simulink model "LinksMotorFahrplan"  (R2012b)
settings: Solver=FixedStepDiscrete  StartTime=0.0  StopTime=25  RelTol=1e-3
libraries: commutil2 x12, c280xlib x3, idelinklib_tgtpref x2, c2833xlib x1
settings Model: Creator=mit064  LastModifiedBy=mit064
settings DataIOCC: SaveOutput=off  SaveTime=off
settings OptimizationCC: OptimizeModelRefInitCode=on  LifeSpan=1
settings HardwareCC: ProdBitPerChar=16  ProdBitPerInt=16  ProdBitPerPointer=16  ProdLargestAtomicInteger=Integer  ProdIntDivRoundTo=Zero  ProdEndianess=LittleEndian  ProdWordSize=16  ProdHWDeviceType=Texas Instruments->C2000
settings RTWCC: SystemTargetFile=idelink_ert.tlc  GenerateMakefile=off  TemplateMakefile=none  Description=IDE Link ERT  ProcessScript=idelink_ert_make_rtw_hook
settings CodeAppCC: IgnoreCustomStorageClasses=off

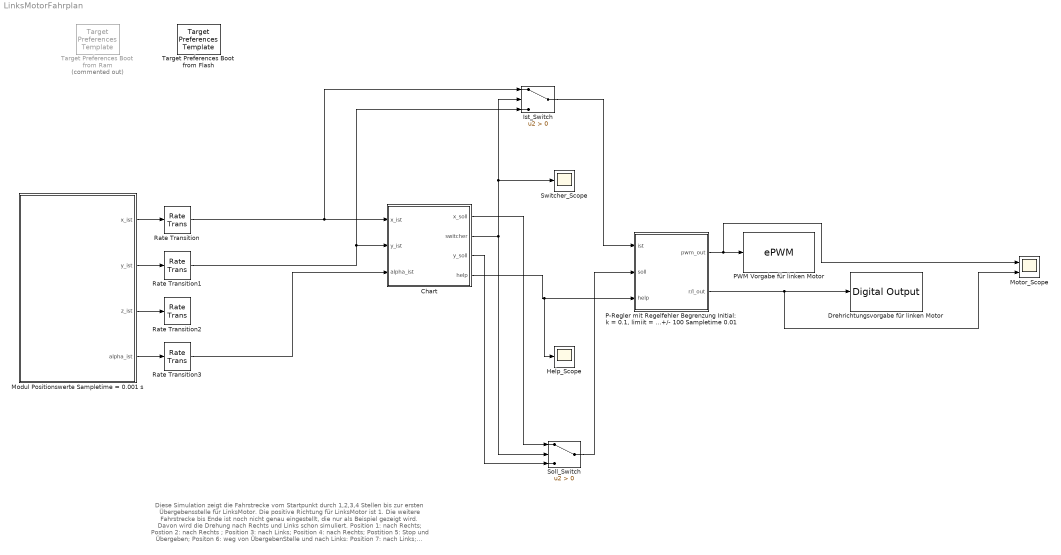
== system LinksMotorFahrplan ==
  note: Diese Simulation zeigt die Fahrstrecke vom Startpunkt durch 1,2,3,4 Stellen bis zur ersten Übergebensstelle für LinksMotor.
      | Die positive Richtung für LinksMotor ist 1.
      | Die weitere Fahrstrecke bis Ende ist noch nicht genau eingestellt, die nur als Beispiel gezeigt wird.
      | Davon wird die Drehung nach Rechts und Links schon simuliert.
      |
      | Position 1: nach Rechts; Postion 2: nach Rechts ; Position 3: nach Links; Position 4: nach Rechts;
      |  Postition 5: Stop und Übergeben; Positon 6: weg von ÜbergebenStelle und nach Links:
      | Position 7: nach Links; Postition 8: nach Links; Position 9: nach Links; Position 10 nach Links
      | Position 11: Stop und Übergeben, Position 12 Stop und Ende
      |
      | Prinzip der Chart:
      | 1. Eingänge: die x_ist, y_ist,alpha_ist Werte werden vom Nexoner Sensor ausgelesen.
      | Durch den Parameter Switcher nimmt der P-Regler die benötige x oder y Werte an.
      | 2. Ausgänge: Durch die Parameter Switcher nimmt ebenfalls der P-Regler die benötige x oder y Werte an.
      | 3. Parameter help in Ausgang: im Fall wenn der Fahrzeug sich nach Links umdrehen will, und  y_soll oder x_soll werte kleiner als den letzen Stelle ist,
      | wird "help" gleich eins, somit dreht sich der Linksmotor in negative Richtung .
      | 4. Parameter help in P-Regler: wenn help gleich eins ist, wird der Motor sich  immer in eine Richtung drehen.
  Chart : Stateflow chart  TreatAsAtomicUnit=on
  Drehrichtungsvorgabe für linken Motor : c2833xlib/Digital Output  GPIO_Number=GPIO16~GPIO23  GPIO_Bit0=off  GPIO_BIT0_Toggle=off  GPIO_Bit1=off  GPIO_BIT1_Toggle=off  GPIO_Bit2=off  GPIO_BIT2_Toggle=off  GPIO_Bit3=off  GPIO_BIT3_Toggle=off  GPIO_Bit4=off  GPIO_BIT4_Toggle=off  GPIO_Bit5=on  GPIO_BIT5_Toggle=off  GPIO_Bit6=off  GPIO_BIT6_Toggle=off  GPIO_Bit7=off  GPIO_BIT7_Toggle=off
  Help_Scope : Scope
  Ist_Switch : Switch  Criteria=u2 > Threshold
  Modul Positionswerte Sampletime = 0.001 s : Subsystem
  Motor_Scope : Scope  NumInputPorts=2
      settings: YMin=-5~-5  YMax=5~5  SaveName=ScopeData2
  "P-Regler mit Regelfehler Begrenzung Initial: k = 0.1, limiit = +/- 100 Sampletime 0.01" : Subsystem
  "PWM Vorgabe für linken Motor " : c280xlib/ePWM  checkMode=off  useModule=ePWM2  periodUnits=Clock cycles  timerSource=Specify via dialog  timerPeriod_clk=64000  timerPeriod_sec=0.0001  countingMode=Up  synchronizationOption=Disable  synchronizationEnable=off  phaseActiveEnable=Disable  phaseDirection=Count down after sync  phaseActive=0  clockPrescale=1  HSclockPrescale=1  ePWMxAStatus=off  CMPAUnits=Clock cycles  CMPASource=Specify via dialog  CMPAValue_per=50  CMPAValue_clk=32000  ePWMxAactionLogic1=Do nothing  ePWMxAactionLogic2=Clear  ePWMxAactionLogic3=Set  ePWMxAactionLogic4=Do nothing  ePWMxAactionLogic5=Do nothing  ePWMxAactionLogic6=Do nothing  ePWMxALoadMode=Load on CTR=Zero  ePWMxACSFenable=off  ePWMxACSFvalue=Forcing Disable  ePWMxASFreload=Zero  enHRPWM=off  HRPWM_LoadMode=CTR=ZERO  HRPWM_CTLMode=Phase control mode  HRPWM_EDGMode=Both edge  enSFO=on  ePWMxBStatus=on  CMPBUnits=Percentages  CMPBSource=Input port  CMPBValue_per=0  CMPBValue_clk=32000  ePWMxBactionLogic1=Do nothing  ePWMxBactionLogic2=Set  ePWMxBactionLogic3=Do nothing  ePWMxBactionLogic4=Do nothing  ePWMxBactionLogic5=Clear  ePWMxBactionLogic6=Do nothing  ePWMxBLoadMode=Load on CTR=Zero  ePWMxBCSFenable=off  ePWMxBCSFvalue=Forcing Disable  ePWMxBSFreload=Zero  enableDBePWMxA=off  enableDBePWMxB=off  DBpolarity=AH  DBedgeDelay=Positive  DBSource_ePWMxA=ePWMxA  DBSource_ePWMxB=ePWMxA  DBperiodSource=Specify via dialog  REDperiod=0  FEDperiod=0  adcstartModuleA=off  adcrequestEventA=First event  adcstartEventA=CTR=Zero  adcstartModuleB=off  adcrequestEventB=First event  adcstartEventB=CTR=Zero  intEn=off  intPrd=First event  intSel=CTR=Zero  chopperEnable=off  chopperFrequency=1  chopperFirstwidth=1  chopperDuty=12.5%  tripZonesource=Specify via dialog  tzselOSHT1=off  tzselOSHT2=off  tzselOSHT3=off  tzselOSHT4=off  tzselOSHT5=off  tzselOSHT6=off  tzselCBC1=off  tzselCBC2=off  tzselCBC3=off  tzselCBC4=off  tzselCBC5=off  tzselCBC6=off  enTzOstIntr=off  enTzCbcIntr=off  ePWMxAforced=No action  ePWMxBforced=No action  timerPeriod=-1  ePWMxAValue=0  ePWMxBValue=0  tripZoneoption=OSHT
  Rate Transition{,1..3} (4 alike) : RateTransition  OutPortSampleTime=0.01
  Soll_Switch : Switch  Criteria=u2 > Threshold
  Switcher_Scope : Scope
  Target Preferences Boot from Flash : idelinklib_tgtpref/Target Preferences Template  Tag=ccslinktgtpref_ccsv4  library=off
  Target Preferences Boot from Ram : idelinklib_tgtpref/Target Preferences Template  Tag=ccslinktgtpref_ccsv4  Commented=on  library=off
  wires:
  "P-Regler mit Regelfehler Begrenzung Initial: k = 0.1, limiit = +/- 100 Sampletime 0.01"/2(r/l_out) -> Motor_Scope/2, Drehrichtungsvorgabe für linken Motor/1
  "P-Regler mit Regelfehler Begrenzung Initial: k = 0.1, limiit = +/- 100 Sampletime 0.01"/1(pwm_out) -> Motor_Scope/1, "PWM Vorgabe für linken Motor "/1
  Ist_Switch/1 -> "P-Regler mit Regelfehler Begrenzung Initial: k = 0.1, limiit = +/- 100 Sampletime 0.01"/1(ist)
  Soll_Switch/1 -> "P-Regler mit Regelfehler Begrenzung Initial: k = 0.1, limiit = +/- 100 Sampletime 0.01"/2(soll)
  Chart/2(switcher) -> Soll_Switch/2, Switcher_Scope/1, Ist_Switch/2
  Chart/1(x_soll) -> Soll_Switch/1
  Chart/3(y_soll) -> Soll_Switch/3
  Chart/4(help) -> Help_Scope/1, "P-Regler mit Regelfehler Begrenzung Initial: k = 0.1, limiit = +/- 100 Sampletime 0.01"/3(help)
  Rate Transition/1 -> Chart/1(x_ist), Ist_Switch/1
  Rate Transition1/1 -> Chart/2(y_ist), Ist_Switch/3
  Rate Transition3/1 -> Chart/3(alpha_ist)
  Modul Positionswerte Sampletime = 0.001 s/1(x_ist) -> Rate Transition/1
  Modul Positionswerte Sampletime = 0.001 s/4(alpha_ist) -> Rate Transition3/1
  Modul Positionswerte Sampletime = 0.001 s/3(z_ist) -> Rate Transition2/1
  Modul Positionswerte Sampletime = 0.001 s/2(y_ist) -> Rate Transition1/1

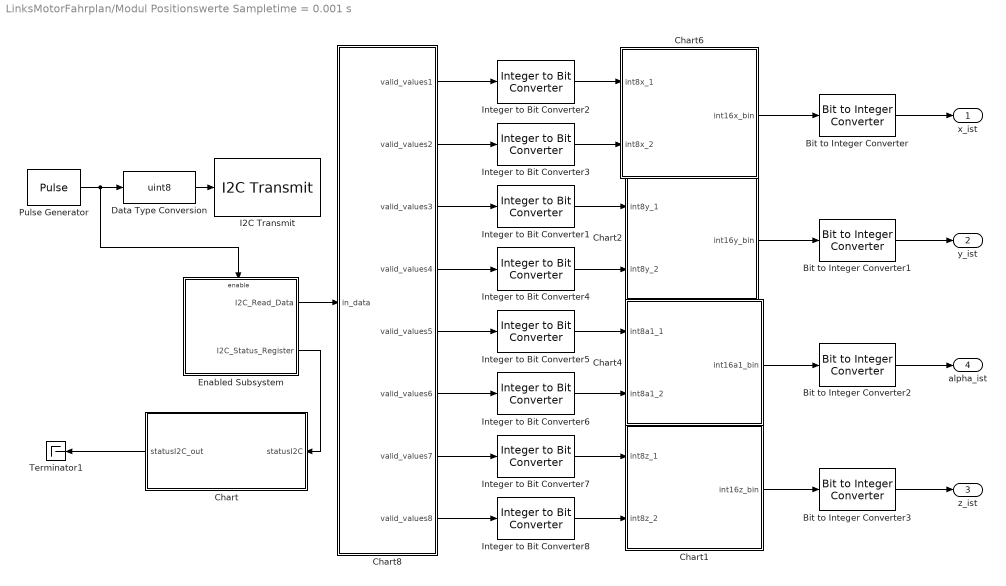
== system LinksMotorFahrplan/Modul Positionswerte Sampletime = 0.001 s ==
  Bit to Integer Converter{,1..3} (4 alike) : commutil2/Bit to Integer Converter  nbits=16  bitOrder=MSB first  signedOutputValues=Signed  outDtype=Inherit via internal rule  outDtypeSigned=Inherit via internal rule
  Chart : Stateflow chart  TreatAsAtomicUnit=on
  Chart1 : Stateflow chart  TreatAsAtomicUnit=on
  Chart2 : Stateflow chart  TreatAsAtomicUnit=on
  Chart4 : Stateflow chart  TreatAsAtomicUnit=on
  Chart6 : Stateflow chart  TreatAsAtomicUnit=on
  Chart8 : Stateflow chart  TreatAsAtomicUnit=on
  Data Type Conversion : DataTypeConversion  OutDataTypeStr=uint8
  Enabled Subsystem : Subsystem  TreatAsAtomicUnit=on
  I2C Transmit : c280xlib/I2C Transmit  addrFormat=7-Bit addressing  saSource=Specify via dialog  SAR=80  bitCount=8  STP=off  RM=off  STR=off
  Integer to Bit Converter{1..8} (8 alike) : commutil2/Integer to Bit Converter  nbits=8  signedInputValues=Unsigned  bitOrder=MSB first  outDtype=uint8
  Pulse Generator : DiscretePulseGenerator  Period=250  PulseWidth=249  SampleTime=0.001
  Terminator1 : Terminator
  x_ist : Outport
  y_ist : Outport  Port=2
  z_ist : Outport  Port=3
  alpha_ist : Outport  Port=4
  wires:
  Chart8/5(valid_values5) -> Integer to Bit Converter5/1
  Chart8/2(valid_values2) -> Integer to Bit Converter3/1
  Chart8/4(valid_values4) -> Integer to Bit Converter4/1
  Chart2/1(int16y_bin) -> Bit to Integer Converter1/1
  Chart8/1(valid_values1) -> Integer to Bit Converter2/1
  Chart8/3(valid_values3) -> Integer to Bit Converter1/1
  Integer to Bit Converter3/1 -> Chart6/2(int8x_2)
  Chart6/1(int16x_bin) -> Bit to Integer Converter/1
  Integer to Bit Converter1/1 -> Chart2/1(int8y_1)
  Integer to Bit Converter2/1 -> Chart6/1(int8x_1)
  Integer to Bit Converter4/1 -> Chart2/2(int8y_2)
  Bit to Integer Converter1/1 -> y_ist/1
  Integer to Bit Converter5/1 -> Chart4/1(int8a1_1)
  Integer to Bit Converter6/1 -> Chart4/2(int8a1_2)
  Bit to Integer Converter/1 -> x_ist/1
  Bit to Integer Converter2/1 -> alpha_ist/1
  Chart8/6(valid_values6) -> Integer to Bit Converter6/1
  Chart4/1(int16a1_bin) -> Bit to Integer Converter2/1
  Chart1/1(int16z_bin) -> Bit to Integer Converter3/1
  Enabled Subsystem/1(I2C_Read_Data) -> Chart8/1(in_data)
  Bit to Integer Converter3/1 -> z_ist/1
  Chart8/8(valid_values8) -> Integer to Bit Converter8/1
  Chart8/7(valid_values7) -> Integer to Bit Converter7/1
  Integer to Bit Converter8/1 -> Chart1/2(int8z_2)
  Integer to Bit Converter7/1 -> Chart1/1(int8z_1)
  Enabled Subsystem/2(I2C_Status_Register) -> Chart/1(statusI2C)
  Chart/1(statusI2C_out) -> Terminator1/1
  Pulse Generator/1 -> Enabled Subsystem/Enable, Data Type Conversion/1
  Data Type Conversion/1 -> I2C Transmit/1

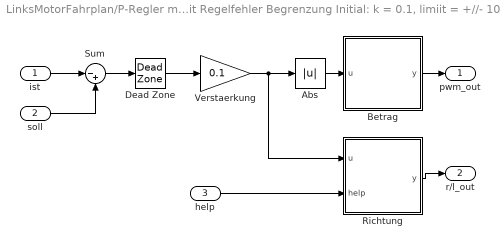
== system LinksMotorFahrplan/P-Regler mit Regelfehler Begrenzung Initial: k = 0.1, limiit = +//- 100 Sampletime 0.01 ==
  ist : Inport
  soll : Inport  Port=2
  help : Inport  Port=3
  Abs : Abs  SampleTime=0.01
  Betrag : MATLAB Function  TreatAsAtomicUnit=on  SystemSampleTime=0.01
  Dead Zone : DeadZone  LowerValue=-100  UpperValue=100  SampleTime=0.01  SaturateOnIntegerOverflow=on
  Richtung : MATLAB Function  TreatAsAtomicUnit=on  SystemSampleTime=0.01
  Sum : Sum  Inputs=|-+  SampleTime=0.01
  Verstaerkung : Gain  Gain=0.1  SampleTime=0.01
  pwm_out : Outport
  r/l_out : Outport  Port=2
  wires:
  Betrag/1(y) -> pwm_out/1
  Sum/1 -> Dead Zone/1
  Verstaerkung/1 -> Abs/1, Richtung/1(u)
  Dead Zone/1 -> Verstaerkung/1
  Abs/1 -> Betrag/1(u)
  soll/1 -> Sum/2
  Richtung/1(y) -> r/l_out/1
  ist/1 -> Sum/1
  help/1 -> Richtung/2(help)

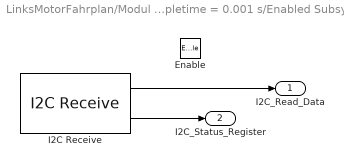
== system LinksMotorFahrplan/Modul Positionswerte Sampletime = 0.001 s/Enabled Subsystem ==
  Enable : EnablePort  StatesWhenEnabling=reset
  I2C Receive : c280xlib/I2C Receive  addrFormat=7-Bit addressing  saSource=Specify via dialog  SAR=80  bitCount=8  dataLength=10  initValue=0  NACK=on  STP=off  STR=on  sampleTime=0.001  dataType=uint8
  I2C_Read_Data : Outport
  I2C_Status_Register : Outport  Port=2
  wires:
  I2C Receive/2 -> I2C_Status_Register/1
  I2C Receive/1 -> I2C_Read_Data/1

== stateflow chart LinksMotorFahrplan/Modul Positionswerte Sampletime = 0.001 s/Chart1 ==
  state Daten_einlesen
  state x0
  state x1_1
    int16z_bin[0] = int8z_1[0];
    int16z_bin[1] = int8z_1[1];
    int16z_bin[2] = int8z_1[2];
    int16z_bin[3] = int8z_1[3];
    int16z_bin[4] = int8z_1[4];
    int16z_bin[5] = int8z_1[5]
    int16z_bin[6] = int8z_1[6];
    int16z_bin[7] = int8z_1[7];
    int16z_bin[8] = int8z_2[0];
    int16z_bin[9] = int8z_2[1];
    int16z_bin[10] = int8z_2[2];
    int16z_bin[11] = int8z_2[3];
    int16z_bin[12] = int8z_2[4];
    int16z_bin[13] = int8z_2[5]
    int16z_bin[14] = int8z_2[6];
    int16z_bin[15] = int8z_2[7];
  x0 -> Daten_einlesen
  (default) -> x0
  Daten_einlesen -> x1_1
  x1_1 -> Daten_einlesen
  data: int8z_1 input size=8; int8z_2 input size=8; int16z_bin output size=16 =0

== stateflow chart LinksMotorFahrplan/Chart ==
  state Start
  state Position_3
    switcher=0;
    help=1;
    state Position_3
      entry:y_soll=400;
    state Stop
      entry:y_soll=y_ist;
      exit:help=0;
    state Drehen_Linke
      entry:y_soll=0;
      exit:help=0;
    state stop
      entry:y_soll=y_ist;
    (default) -> Position_3.Position_3
    Position_3.Position_3 -> Position_3.Stop : [y_ist<402&&y_ist>398]
    Position_3.Stop -> Position_3.Drehen_Linke : [after(1,sec)]
    Position_3.Drehen_Linke -> Position_3.stop : [alpha_ist<65&&alpha_ist>61]
  state Position_4
    switcher=0;
    help=1;
    state Position_4
      entry:y_soll=700;
    state Stop
      entry:y_soll=y_ist;
    state Drehen_Recht
      entry:y_soll=0;
    state stop
      entry:y_soll=y_ist;
    (default) -> Position_4.Position_4
    Position_4.Position_4 -> Position_4.Stop : [y_ist<702&&y_ist>698]
    Position_4.Stop -> Position_4.Drehen_Recht : [after(1,sec)]
    Position_4.Drehen_Recht -> Position_4.stop : [alpha_ist<-61&&alpha_ist>-65]
  state Position_1
    switcher=0;
    help=1;
    state Position_1
      entry:y_soll=350;
    state Stop
      entry:y_soll=y_ist;
    state Drehen_Recht
      entry:y_soll=0;
    state stop
      entry:y_soll=y_ist;
    (default) -> Position_1.Position_1
    Position_1.Position_1 -> Position_1.Stop : [y_ist<352&&y_ist>348]
    Position_1.Stop -> Position_1.Drehen_Recht : [after(1,sec)]
    Position_1.Drehen_Recht -> Position_1.stop : [alpha_ist<79&&alpha_ist>75]
  state Position_2
    switcher=0;
    help=1;
    state Position_2
      entry:y_soll=900;
    state Stop
      entry:y_soll=y_ist;
    state Drehen_Recht
      entry:y_soll=0;
    state stop
      entry:y_soll=y_ist;
    (default) -> Position_2.Position_2
    Position_2.Position_2 -> Position_2.Stop : [y_ist<902&&y_ist>898]
    Position_2.Stop -> Position_2.Drehen_Recht : [after(1,sec)]
    Position_2.Drehen_Recht -> Position_2.stop : [alpha_ist>-61&&alpha_ist<-57]
  state Position_6
    switcher=0;
    help=1;
    state Position_6
      entry:y_soll=300;
    state Stop
      entry:y_soll=y_ist;
      exit:help=0;
    state Drehen_Linke
      entry:y_soll=0;
      exit:help=0;
    state stop
      entry:y_soll=y_ist;
    (default) -> Position_6.Position_6
    Position_6.Position_6 -> Position_6.Stop : [y_ist<302&&y_ist>298]
    Position_6.Stop -> Position_6.Drehen_Linke : [after(1,sec)]
    Position_6.Drehen_Linke -> Position_6.stop : [alpha_ist<-32&&alpha_ist>-36]
  state Position_5_give
    switcher=0;
    help=1;
    state Position_5
      entry:y_soll=400;
    state Stop
      entry:y_soll=y_ist;
    state Drehen_Recht
      entry:y_soll=0;
    state stop
      entry:y_soll=y_ist;
    (default) -> Position_5
    Position_5 -> Position_5_give.Stop : [y_ist<402&&y_ist>398]
    Position_5_give.Stop -> Position_5_give.Drehen_Recht : [after(5,sec)]
    Position_5_give.Drehen_Recht -> Position_5_give.stop : [alpha_ist<-88]
  state Position_7
    switcher=1;
    help=1;
    state Position_7
      entry:x_soll=1400;
    state Stop
      entry:x_soll=x_ist;
      exit:help=0;
    state Drehen_Linke
      entry:x_soll=0;
      exit:help=0;
    state stop
      entry:x_soll=x_ist;
    (default) -> Position_7.Position_7
    Position_7.Position_7 -> Position_7.Stop : [x_ist<1402&&x_ist>1398]
    Position_7.Stop -> Position_7.Drehen_Linke : [after(1,sec)]
    Position_7.Drehen_Linke -> Position_7.stop : [alpha_ist<47&&alpha_ist>43]
  state Position_8
    switcher=1;
    help=1;
    state Position_8
      entry:x_soll=1700;
    state Stop
      entry:x_soll=x_ist;
      exit:help=0;
    state Drehen_Linke
      entry:x_soll=0;
      exit:help=0;
    state stop
      entry:x_soll=x_ist;
    (default) -> Position_8.Position_8
    Position_8.Position_8 -> Position_8.Stop : [x_ist<1702&&x_ist>1698]
    Position_8.Stop -> Position_8.Drehen_Linke : [after(1,sec)]
    Position_8.Drehen_Linke -> Position_8.stop : [alpha_ist<47&&alpha_ist>43]
  state Position_11_give
    switcher=0;
    help=1;
    state Position_11
      entry:y_soll=300;
    state Stop
      entry:y_soll=y_ist;
    (default) -> Position_11
    Position_11 -> Position_11_give.Stop : [y_ist<302&&y_ist>298]
  state Position_12_End
    switcher=0;
    help=1;
    state Position_12
      entry:y_soll=-200;
    state Stop
      entry:y_soll=y_ist;
    (default) -> Position_12
    Position_12 -> Position_12_End.Stop : [y_ist<-198&&y_ist>-202]
  state Position_9
    switcher=1;
    help=1;
    state Position_9
      entry:x_soll=1100;
    state Stop
      entry:x_soll=x_ist;
      exit:help=0;
    state Drehen_Linke
      entry:x_soll=0;
      exit:help=0;
    state stop
      entry:x_soll=x_ist;
    (default) -> Position_9.Position_9
    Position_9.Position_9 -> Position_9.Stop : [x_ist<1102&&x_ist>1098]
    Position_9.Stop -> Position_9.Drehen_Linke : [after(1,sec)]
    Position_9.Drehen_Linke -> Position_9.stop : [alpha_ist<2&&alpha_ist>-2]
  state Position_10
    switcher=0;
    help=1;
    state Position_10
      entry:y_soll=300;
    state Stop
      entry:y_soll=y_ist;
      exit:help=0;
    state Drehen_Linke
      entry:y_soll=0;
      exit:help=0;
    state stop
      entry:y_soll=y_ist;
    (default) -> Position_10.Position_10
    Position_10.Position_10 -> Position_10.Stop : [y_ist<302&&y_ist>298]
    Position_10.Stop -> Position_10.Drehen_Linke : [after(1,sec)]
    Position_10.Drehen_Linke -> Position_10.stop : [alpha_ist<-88]
  (default) -> Start
  Start -> Position_1 : [after(2,sec)]
  Position_3 -> Position_4 : [after(0.5,sec)]
  Position_1 -> Position_2 : [after(0.5,sec)]
  Position_2 -> Position_3 : [after(0.5,sec)]
  Position_4 -> Position_5_give : [after(0.5,sec)]
  Position_7 -> Position_8 : [after(0.5,sec)]
  Position_6 -> Position_7 : [after(0.5,sec)]
  Position_5_give -> Position_6 : [after(0.5,sec)]
  Position_8 -> Position_9 : [after(0.5,sec)]
  Position_11_give -> Position_12_End : [after(5,sec)]
  Position_9 -> Position_10 : [after(0.5,sec)]
  Position_10 -> Position_11_give : [after(0.5,sec)]
  data: x_ist input; y_ist input; alpha_ist input; x_soll output; switcher output; y_soll output; help output

== stateflow chart LinksMotorFahrplan/Modul Positionswerte Sampletime = 0.001 s/Chart2 ==
  state Daten_einlesen
  state x0
  state x1_1
    int16y_bin[0] = int8y_1[0];
    int16y_bin[1] = int8y_1[1];
    int16y_bin[2] = int8y_1[2];
    int16y_bin[3] = int8y_1[3];
    int16y_bin[4] = int8y_1[4];
    int16y_bin[5] = int8y_1[5]
    int16y_bin[6] = int8y_1[6];
    int16y_bin[7] = int8y_1[7];
    int16y_bin[8] = int8y_2[0];
    int16y_bin[9] = int8y_2[1];
    int16y_bin[10] = int8y_2[2];
    int16y_bin[11] = int8y_2[3];
    int16y_bin[12] = int8y_2[4];
    int16y_bin[13] = int8y_2[5]
    int16y_bin[14] = int8y_2[6];
    int16y_bin[15] = int8y_2[7];
  x0 -> Daten_einlesen
  (default) -> x0
  Daten_einlesen -> x1_1
  x1_1 -> Daten_einlesen
  data: int8y_1 input size=8; int8y_2 input size=8; int16y_bin output size=16 =0

== matlab function LinksMotorFahrplan/P-Regler mit Regelfehler Begrenzung Initial: k = 0.1, limiit = +//- 100 Sampletime 0.01/Betrag ==
  settings: updateMethod=DISCRETE  sampleTime=0.01
  data: u input; y output
function y = fcn( u )

if 0.5 < u && u < 60
    y = 60;
elseif u <= 0.5
    y = 0;
elseif u >= 100
    y = 100;
else
    y = abs(u);
end

== stateflow chart LinksMotorFahrplan/Modul Positionswerte Sampletime = 0.001 s/Chart4 ==
  state Daten_einlesen
  state x0
  state x1_1
    int16a1_bin[0] = int8a1_1[0];
    int16a1_bin[1] = int8a1_1[1];
    int16a1_bin[2] = int8a1_1[2];
    int16a1_bin[3] = int8a1_1[3];
    int16a1_bin[4] = int8a1_1[4];
    int16a1_bin[5] = int8a1_1[5]
    int16a1_bin[6] = int8a1_1[6];
    int16a1_bin[7] = int8a1_1[7];
    int16a1_bin[8] = int8a1_2[0];
    int16a1_bin[9] = int8a1_2[1];
    int16a1_bin[10] = int8a1_2[2];
    int16a1_bin[11] = int8a1_2[3];
    int16a1_bin[12] = int8a1_2[4];
    int16a1_bin[13] = int8a1_2[5]
    int16a1_bin[14] = int8a1_2[6];
    int16a1_bin[15] = int8a1_2[7];
  x0 -> Daten_einlesen
  (default) -> x0
  Daten_einlesen -> x1_1
  x1_1 -> Daten_einlesen
  data: int8a1_1 input size=8; int8a1_2 input size=8; int16a1_bin output size=16 =0

== matlab function LinksMotorFahrplan/P-Regler mit Regelfehler Begrenzung Initial: k = 0.1, limiit = +//- 100 Sampletime 0.01/Richtung ==
  settings: updateMethod=DISCRETE  sampleTime=0.01
  data: u input; y output; help input
function y = fcn( u,help) 

if u > 0
    y = 1;
else
    y = 0+help;
end

== stateflow chart LinksMotorFahrplan/Modul Positionswerte Sampletime = 0.001 s/Chart6 ==
  state Daten_einlesen
  state x0
  state x1_1
    int16x_bin[0] = int8x_1[0];
    int16x_bin[1] = int8x_1[1];
    int16x_bin[2] = int8x_1[2];
    int16x_bin[3] = int8x_1[3];
    int16x_bin[4] = int8x_1[4];
    int16x_bin[5] = int8x_1[5]
    int16x_bin[6] = int8x_1[6];
    int16x_bin[7] = int8x_1[7];
    int16x_bin[8] = int8x_2[0];
    int16x_bin[9] = int8x_2[1];
    int16x_bin[10] = int8x_2[2];
    int16x_bin[11] = int8x_2[3];
    int16x_bin[12] = int8x_2[4];
    int16x_bin[13] = int8x_2[5]
    int16x_bin[14] = int8x_2[6];
    int16x_bin[15] = int8x_2[7];
  x0 -> Daten_einlesen
  (default) -> x0
  Daten_einlesen -> x1_1
  x1_1 -> Daten_einlesen
  data: int8x_1 input size=8; int8x_2 input size=8; int16x_bin output size=16 =0

== stateflow chart LinksMotorFahrplan/Modul Positionswerte Sampletime = 0.001 s/Chart8 ==
  state init
    values_out1[0] = 0;
    values_out1[1] = 0;
    values_out1[2] = 0;
    values_out1[3] = 0;
    values_out1[4] = 0;
    values_out1[5] = 0;
    values_out1[6] = 0;
    values_out1[7] = 0;
    values_out1[8] = 0;
    values_out1[9] = 0;
    values_out1[10] = 0;
    values_out1[11] = 0;
    values_out1[12] = 0;
    values_out1[13] = 0;
    values_out1[14] = 0;
    values_out1[15] = 0;
    values_out1[16] = 0;
    values_out1[17] = 0;
    values_out1[18] = 0;
    values_out1[19] = 0;
  state wert_erkannt
    values_out1[0] = in_data[0];
    values_out1[1] = in_data[1];
    values_out1[2] = in_data[2];
    values_out1[3] = in_data[3];
    values_out1[4] = in_data[4];
    values_out1[5] = in_data[5];
    values_out1[6] = in_data[6];
    values_out1[7] = in_data[7];
    values_out1[8] = in_data[8];
    values_out1[9] = in_data[9];
  state Anfang_found_Schritt_uebertragen_weglassen_performance
    x_found = x_found +1;
  state x5_valid_data_found1
    valid_values1 = values_out1[search+1];
    valid_values2 = values_out1[search+2];
    valid_values3 = values_out1[search+3];
    valid_values4 = values_out1[search+4];
    valid_values5 = values_out1[search+5];
    valid_values6 = values_out1[search+6];
    valid_values7 = values_out1[search+7];
    valid_values8 = values_out1[search+8];
    zaehler = zaehler +1;
  state wert_erkannt2
    values_out1[10] = in_data[0];
    values_out1[11] = in_data[1];
    values_out1[12] = in_data[2];
    values_out1[13] = in_data[3];
    values_out1[14] = in_data[4];
    values_out1[15] = in_data[5];
    values_out1[16] = in_data[6];
    values_out1[17] = in_data[7];
    values_out1[18] = in_data[8];
    values_out1[19] = in_data[9];
    search = 0;
    counter = counter + 1;
  state x1_search1
    search = search + 1;
  x5_valid_data_found1 -> wert_erkannt
  x1_search1 -> wert_erkannt [order 3]
  init -> wert_erkannt
  (default) -> init
  Anfang_found_Schritt_uebertragen_weglassen_performance -> x5_valid_data_found1 [order 1] : [((values_out1[search]+values_out1[search+1]+values_out1[search+2]+values_out1[search+3]+values_out1[search+4]+values_out1[search+5]+values_out1[search+6]+values_out1[search+7]+values_out1[search+8])) == values_out1[search+9]]
  wert_erkannt -> wert_erkannt2
  Anfang_found_Schritt_uebertragen_weglassen_performance -> x5_valid_data_found1 [order 2] : [((values_out1[search]+values_out1[search+1]+values_out1[search+2]+values_out1[search+3]+values_out1[search+4]+values_out1[search+5]+values_out1[search+6]+values_out1[search+7]+values_out1[search+8])-(256)) == values_out1[search+9]]
  Anfang_found_Schritt_uebertragen_weglassen_performance -> x5_valid_data_found1 [order 3] : [((values_out1[search]+values_out1[search+1]+values_out1[search+2]+values_out1[search+3]+values_out1[search+4]+values_out1[search+5]+values_out1[search+6]+values_out1[search+7]+values_out1[search+8])-(512)) == values_out1[search+9]]
  Anfang_found_Schritt_uebertragen_weglassen_performance -> x5_valid_data_found1 [order 7] : [((values_out1[search]+values_out1[search+1]+values_out1[search+2]+values_out1[search+3]+values_out1[search+4]+values_out1[search+5]+values_out1[search+6]+values_out1[search+7]+values_out1[search+8])-(768)) == values_out1[search+9]]
  Anfang_found_Schritt_uebertragen_weglassen_performance -> x5_valid_data_found1 [order 6] : [((values_out1[search]+values_out1[search+1]+values_out1[search+2]+values_out1[search+3]+values_out1[search+4]+values_out1[search+5]+values_out1[search+6]+values_out1[search+7]+values_out1[search+8])-(1024)) == values_out1[search+9]]
  Anfang_found_Schritt_uebertragen_weglassen_performance -> x5_valid_data_found1 [order 5] : [((values_out1[search]+values_out1[search+1]+values_out1[search+2]+values_out1[search+3]+values_out1[search+4]+values_out1[search+5]+values_out1[search+6]+values_out1[search+7]+values_out1[search+8])-(1280)) == values_out1[search+9]]
  Anfang_found_Schritt_uebertragen_weglassen_performance -> x5_valid_data_found1 [order 4] : [((values_out1[search]+values_out1[search+1]+values_out1[search+2]+values_out1[search+3]+values_out1[search+4]+values_out1[search+5]+values_out1[search+6]+values_out1[search+7]+values_out1[search+8])-(1536)) == values_out1[search+9]]
  Anfang_found_Schritt_uebertragen_weglassen_performance -> x5_valid_data_found1 [order 8] : [((values_out1[search]+values_out1[search+1]+values_out1[search+2]+values_out1[search+3]+values_out1[search+4]+values_out1[search+5]+values_out1[search+6]+values_out1[search+7]+values_out1[search+8])-(1792)) == values_out1[search+9]]
  Anfang_found_Schritt_uebertragen_weglassen_performance -> x5_valid_data_found1 [order 10] : [((values_out1[search]+values_out1[search+1]+values_out1[search+2]+values_out1[search+3]+values_out1[search+4]+values_out1[search+5]+values_out1[search+6]+values_out1[search+7]+values_out1[search+8])-(2048)) == values_out1[search+9]]
  Anfang_found_Schritt_uebertragen_weglassen_performance -> x1_search1 [order 9]
  wert_erkannt2 -> Anfang_found_Schritt_uebertragen_weglassen_performance [order 1] : [values_out1[search] == 88]
  x1_search1 -> Anfang_found_Schritt_uebertragen_weglassen_performance [order 1] : [values_out1[search] == 88]
  wert_erkannt2 -> x1_search1 [order 2]
  x1_search1 -> x1_search1 [order 2] : [search < 19]
  data: in_data input size=10; values_out1 local int16 size=20; zaehler local int32 =0; search local int16; valid_values1 output int16 size=1; valid_values2 output int16 size=1; valid_values3 output int16 size=1; valid_values4 output int16 size=1; valid_values5 output int16 size=1; valid_values6 output int16 size=1; valid_values7 output int16 size=1; valid_values8 output int16 size=1; counter local int32 =0; x_found local int32 =0

== stateflow chart LinksMotorFahrplan/Modul Positionswerte Sampletime = 0.001 s/Chart ==
  state x1
    statusI2C_out = statusI2C;
  x1 -> x1
  (default) -> x1
  data: statusI2C input; statusI2C_out output
